simulink model "RT_ss2011_A4"  (R2013a)
settings: Solver=ode45  StartTime=0.0  StopTime=10.0  RelTol=1e-3
values from neighbouring files (symbols this model uses):
  ClosedLoop = 0    [RT_klausurvorb.m]
  ps = tf(1,[1 1 0])    [RT_Klausur_SS2014.m]    (also in RT_klausurvorb.m = pole(g0))
  qs = tf(10,[1 20])    [RT_Klausur_SS2014.m]    (also in RT_klausurvorb.m = tf(1,[0.05 1]))
libraries: simulink x1
settings Model: Creator=mainster  LastModifiedBy=mainster
settings DebuggingCC: SolverPrmCheckMsg=none

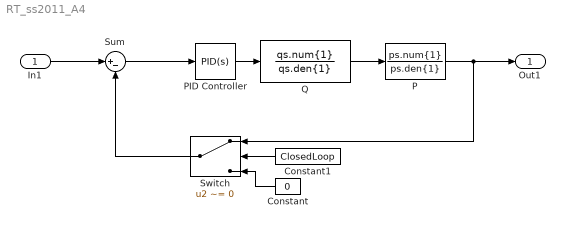
== system RT_ss2011_A4 ==
  In1 : Inport
  Constant : Constant  Value=0
  Constant1 : Constant  Value=ClosedLoop
  P : TransferFcn  Numerator=ps.num{1}  Denominator=ps.den{1}
  PID Controller : simulink/Continuous/PID Controller  Controller=PID  TimeDomain=Continuous-time  SampleTime=1  IntegratorMethod=Forward Euler  FilterMethod=Forward Euler  Form=Parallel  P=2.4448994087806  I=0.0425571888411145  D=1.63931663994462  N=5.44844684216306  InitialConditionSource=internal  InitialConditionForIntegrator=0  InitialConditionForFilter=0  ExternalReset=none  LimitOutput=off  UpperSaturationLimit=inf  LowerSaturationLimit=-inf  LinearizeAsGain=on  AntiWindupMode=none  Kb=1  TrackingMode=off  Kt=1  PParamMin=[]  PParamMax=[]  IParamMin=[]  IParamMax=[]  DParamMin=[]  DParamMax=[]  NParamMin=[]  NParamMax=[]  KbParamMin=[]  KbParamMax=[]  KtParamMin=[]  KtParamMax=[]  POutMin=[]  POutMax=[]  IOutMin=[]  IOutMax=[]  DOutMin=[]  DOutMax=[]  NOutMin=[]  NOutMax=[]  KbOutMin=[]  KbOutMax=[]  KtOutMin=[]  KtOutMax=[]  IntegratorOutMin=[]  IntegratorOutMax=[]  FilterOutMin=[]  FilterOutMax=[]  SumOutMin=[]  SumOutMax=[]  SumI1OutMin=[]  SumI1OutMax=[]  SumI2OutMin=[]  SumI2OutMax=[]  SumI3OutMin=[]  SumI3OutMax=[]  SumDOutMin=[]  SumDOutMax=[]  SaturationOutMin=[]  SaturationOutMax=[]  IntegratorContinuousStateAttributes=''  IntegratorStateMustResolveToSignalObject=off  IntegratorRTWStateStorageClass=Auto  FilterContinuousStateAttributes=''  FilterStateMustResolveToSignalObject=off  FilterRTWStateStorageClass=Auto
  "Q " : TransferFcn  Numerator=qs.num{1}  Denominator=qs.den{1}
  Sum : Sum  Inputs=|+-
  Switch : Switch  Criteria=u2 ~= 0
  Out1 : Outport
  wires:
  PID Controller/1 -> "Q "/1
  "Q "/1 -> P/1
  P/1 -> Switch/1, Out1/1
  In1/1 -> Sum/1
  Sum/1 -> PID Controller/1
  Switch/1 -> Sum/2
  Constant/1 -> Switch/3
  Constant1/1 -> Switch/2
